simulink model "zadanie1_sim"  (R2025a)
settings: Solver=VariableStepAuto  StartTime=0.0  StopTime=10.0  RelTol=1e-3
values from neighbouring files (symbols this model uses):
  A = [0 1 0 ... (first row only)    [zadanie1.m]    (also in zadanie2.m = [0  1  0 0)
  B = [0 ... (first row only)    [zadanie1.m]    (also in zadanie2.m)
  C = [1 0 0]    [zadanie1.m]    (also in zadanie2.m = [1 0 0 0])
  D = 0    [zadanie1.m]    (also in zadanie2.m)
settings Model: Creator=D106-Student  LastModifiedBy=Dejmian

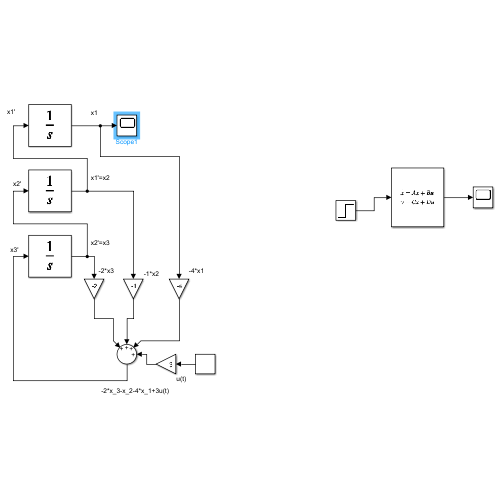
[thumbnail: Simulink's stored preview of the top-level diagram]
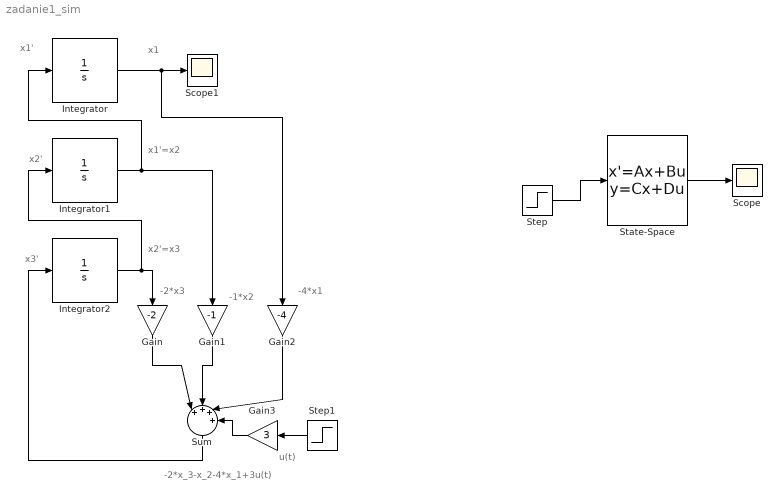
== system zadanie1_sim ==
  note: u(t)
  note: -2*x_3-x_2-4*x_1+3u(t)
  note: x3'
  note: -4*x1
  note: -1*x2
  note: -2*x3
  note: x2'=x3
  note: x2'
  note: x1'=x2
  note: x1'
  note: x1
  Gain : Gain  Gain=-2
  Gain1 : Gain  Gain=-1
  Gain2 : Gain  Gain=-4
  Gain3 : Gain  Gain=3
  Integrator : Integrator
  Integrator1 : Integrator
  Integrator2 : Integrator
  Scope : Scope
      settings: ActiveDisplayYMinimum=-1.0853310544918917  ActiveDisplayYMaximum=3.2308741196767494
  Scope1 : Scope
      settings: ActiveDisplayYMinimum=-1.0853310544918917  ActiveDisplayYMaximum=3.2308741196767494
  State-Space : StateSpace  A=A  B=B  C=C  D=D  InitialCondition=0
  Step : Step  SampleTime=0
  Step1 : Step  SampleTime=0
  Sum : Sum  Inputs=|++++
  wires:
  State-Space/1 -> Scope/1
  Integrator/1 -> Gain2/1, Scope1/1
  Integrator1/1 -> Gain1/1, Integrator/1
  Integrator2/1 -> Gain/1, Integrator1/1
  Gain/1 -> Sum/1
  Gain1/1 -> Sum/2
  Gain2/1 -> Sum/3
  Sum/1 -> Integrator2/1
  Step1/1 -> Gain3/1
  Gain3/1 -> Sum/4
  Step/1 -> State-Space/1
